simulink model "SMES_DC_STEP_1170KW_1000V_0"  (R2020a)
settings: Solver=VariableStepAuto  StartTime=0.0  StopTime=2  RelTol=1e-3
InitFcn:
  | Timer= 1e-3
StartFcn:
  | Timer= 1e-3
undefined symbols (not defined in the file): L
libraries: powerlib x33, simulink x5, powerlib_meascontrol x4
settings Model: Creator=JGC  LastModifiedBy=AGP
settings DataIOCC: ReturnWorkspaceOutputs=off

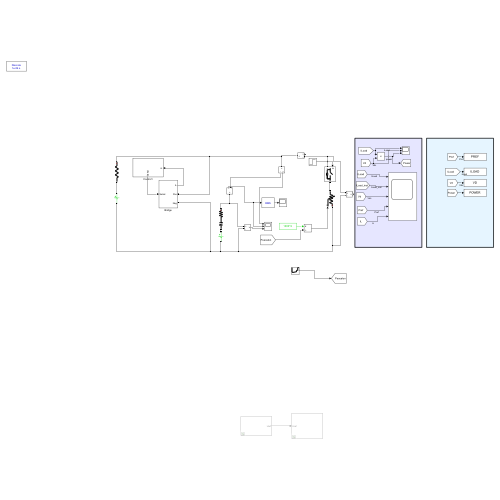
[thumbnail: Simulink's stored preview of the top-level diagram]
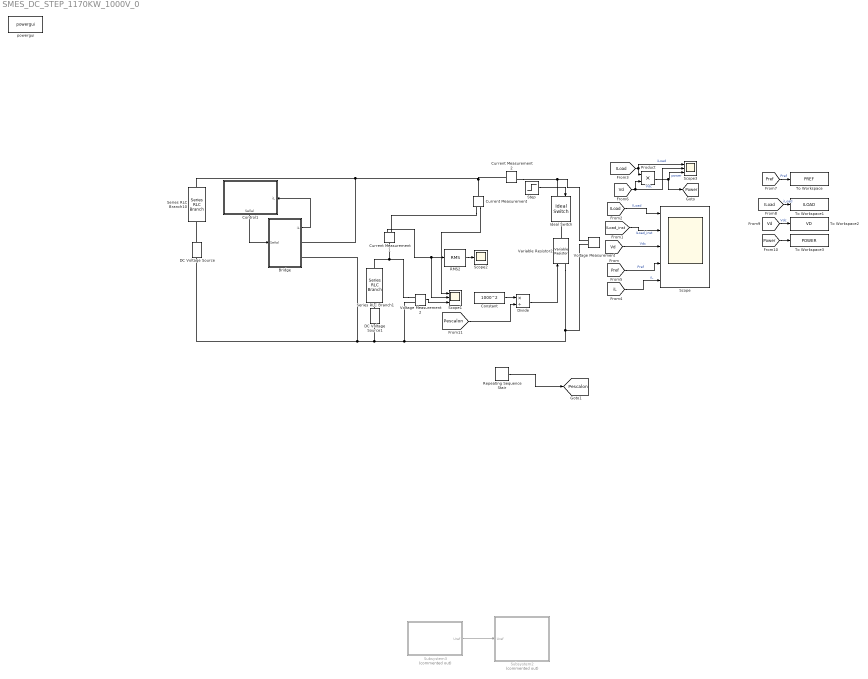
== system SMES_DC_STEP_1170KW_1000V_0 ==
  Bridge : Subsystem
  Constant : Constant  Value=1000^2
  Control1 : Subsystem
      settings: PortSchema="{\"entries\":[{\"content\":{\"sides\":[{\"content\":{},\"type\":\"ConnectorPlacement.EquallySpacedRectSide\",\"uuid\":\"048239fd-db1d-471e-8dcc-44b0bb6d6223\"},{\"content\":{\"connectorIds\":[\"In1\"],\"side\":\"RIGHT\"},\"type\":\"ConnectorPlacement.EquallySpacedRectSide\",\"uuid\":\"9151a5a4-d268-441e-9897-4ef179ef940a\"},{\"content\":{\"side\":\"TOP\"},\"type\":\"ConnectorPlacement.EquallySpacedRectSide\",\"uuid\":\"4fbf07e4-6277-4577-bdb6-c05e0e5af188\"},{\"content\":{\"connectorIds\":[\"Out1\"],\"side\":\"BOTTOM\"},\"type\":\"ConnectorPlacement.EquallySpacedRectSide\",\"uuid\":\"b1bdda97-6966-4786-9e6a-4bb3780cee9c\"}]},\"type\":\"ConnectorPlacement.EquallySpacedConnector\",\"uuid\":\"ea29d1f9-a328-47e5-9b19-c2665d8c639d\"}],\"packageUris\":[\"http://schema.mathworks.com/mf0/Connector/R2020b\"],\"version\":\"1.0\"}"
  Current Measurement : powerlib/Measurements/Current Measurement  PhasorSimulation=off  OutputType=Complex  PSBequivalent=0
  Current Measurement1 : powerlib/Measurements/Current Measurement  PhasorSimulation=off  OutputType=Complex  PSBequivalent=0
  Current Measurement2 : powerlib/Measurements/Current Measurement  PhasorSimulation=off  OutputType=Complex  PSBequivalent=0
  DC Voltage Source : powerlib/Electrical Sources/DC Voltage Source  Amplitude=1000  Measurements=None
  DC Voltage Source1 : powerlib/Electrical Sources/DC Voltage Source  Amplitude=1000  Measurements=None
  Divide : Product  Inputs=*/
  Ideal Switch : powerlib/Power Electronics/Ideal Switch  Ron=0.001  Lon=0  IC=0  Rs=1e5  Cs=inf  Measurements=off
  Product : Product
  RMS2 : powerlib_meascontrol/Measurements/RMS  TrueRMS=on  Freq=50  RMSInit=0  Ts=0
  Repeating Sequence Stair : simulink/Sources/Repeating Sequence Stair  OutValues=[35e3 50e3 100e3 175e3 500e3 1170e3].'  tsamp=0.2  OutMin=[]  OutMax=[]  OutDataTypeStr=double  OutputDataTypeScalingMode=double  OutDataType=fixdt(0,8)  ConRadixGroup=Best Precision: Vector-wise  OutScaling=2^-12
  Scope : Scope  NumInputPorts=5
  Scope1 : Scope  NumInputPorts=3
  Scope2 : Scope
  Scope3 : Scope  NumInputPorts=3
  Series RLC Branch1 : powerlib/Elements/Series RLC Branch  LConnTagsString=__new0  RConnTagsString=__new0  BranchType=RC  Resistance=0.15e-3*200  Inductance=L  SetiL0=off  InitialCurrent=0  Capacitance=3400/200  Setx0=off  InitialVoltage=800  Measurements=None
  Series RLC Branch10 : powerlib/Elements/Series RLC Branch  LConnTagsString=__new0  RConnTagsString=__new0  BranchType=R  Resistance=1e-2  Inductance=L  SetiL0=off  InitialCurrent=0  Capacitance=1e-3  Setx0=off  InitialVoltage=800  Measurements=None
  Step : Step  Time=0.01  SampleTime=0
  Subsystem2 : Subsystem  Commented=on
  Subsystem3 : Subsystem  Commented=on
  To Workspace : ToWorkspace  VariableName=PREF  SaveFormat=Structure With Time  SampleTime=Timer
  To Workspace1 : ToWorkspace  VariableName=ILOAD  SaveFormat=Structure With Time  SampleTime=Timer
  To Workspace2 : ToWorkspace  VariableName=VD  SaveFormat=Structure With Time  SampleTime=Timer
  To Workspace3 : ToWorkspace  VariableName=POWER  SaveFormat=Structure With Time  SampleTime=Timer
  Variable Resistor2 : powerlib/Elements/Variable Resistor  Rabsmin=1e-3
  Voltage Measurement : powerlib/Measurements/Voltage Measurement  PhasorSimulation=off  OutputType=Complex  PSBequivalent=0
  Voltage Measurement2 : powerlib/Measurements/Voltage Measurement  PhasorSimulation=off  OutputType=Complex  PSBequivalent=0
  powergui : powerlib/powergui  Priority=1  SimulationMode=Discrete  SampleTime=1e-6  frequency=60  Iterations=50  frequencyindice=0  Pbase=100e6  ErrMax=1e-4  UnitsV=kV  UnitsW=MW  buscounter=0  FunctionMessages=off  echomessages=off  EnableUseOfTLC=off  CurrentSourceSwitches=off  DisableSnubberDevices=off  DisableRonSwitches=off  DisableVfSwitches=off  DisplayEquations=off  AutomaticDiscreteSolvers=off  SolverType=Tustin/Backward Euler (TBE)  Interpol=off  ExternalGateDelay=off  methode=off  Ts=100  x0status=zero  SPID=off  SwTol=0  HookPort=off  NonlinearTolerance=1e-4  nMaxIteration=100  ContinueOnMaxIteration=off  RestoreLinks=warning  ResistiveCurrentMeasurement=off  Frange=[0:2:500]  Ylog=off  Xlog=on  ShowGrid=off  save=off  variable=ZData  structure=0  ZoomFFT=off  StartTime=0.0  cycles=1  DisplayStyle=1  fundamental=60  FreqAxis=off  MaxFrequency=1000  frequencyindicesteady=1  RmsSteady=1  display=off
  tag scope: Pescalon=global, Power=global
  wires:
  Step/1 -> Ideal Switch/1
  [Pref] -> Scope/4  "Pref"
  Current Measurement/1 -> Scope1/1
  Subsystem3/1(Uref) -> Subsystem2/1(Uref)
  [iL] -> Scope/5  "iL"
  [ILoad_inst] -> Scope/2  "ILoad_inst"
  [ILoad] -> Scope/1  "ILoad"
  [Vd] -> Scope/3  "Vdc"
  Control1/1("Señal ") -> Bridge/1(Señal)
  Bridge/1(iL) -> Control1/1(iL)
  Current Measurement1/1 -> Scope1/2, RMS2/1
  Voltage Measurement2/1 -> Scope1/3
  RMS2/1 -> Scope2/1
  [Pescalon] -> Divide/2
  Divide/1 -> Variable Resistor2/1
  Constant/1 -> Divide/1
  [ILoad] -> Product/1, Scope3/1  "iLoad"
  Product/1 -> [Power], Scope3/3  "power"
  [Vd] -> Product/2, Scope3/2  "Vdc"
  [Pref] -> To Workspace/1  "Pref"
  [ILoad] -> To Workspace1/1  "iLoad"
  [Vd] -> To Workspace2/1  "Vdc"
  [Power] -> To Workspace3/1
  Repeating Sequence Stair/1 -> [Pescalon]
  connections:
  DC Voltage Source/RConn1 -- Series RLC Branch10/RConn1
  Current Measurement/RConn1 -- Current Measurement1/RConn1
  Variable Resistor2/RConn1 -- Ideal Switch/RConn1
  Ideal Switch/LConn1 -- Current Measurement2/RConn1 -- Voltage Measurement/LConn1
  Bridge/RConn2 -- DC Voltage Source/LConn1 -- DC Voltage Source1/LConn1 -- Voltage Measurement/LConn2 -- Variable Resistor2/LConn1 -- Voltage Measurement2/LConn2
  Voltage Measurement2/LConn1 -- Series RLC Branch1/LConn1 -- Current Measurement1/LConn1
  DC Voltage Source1/RConn1 -- Series RLC Branch1/RConn1
  Current Measurement/LConn1 -- Current Measurement2/LConn1 -- Bridge/RConn1 -- Series RLC Branch10/LConn1

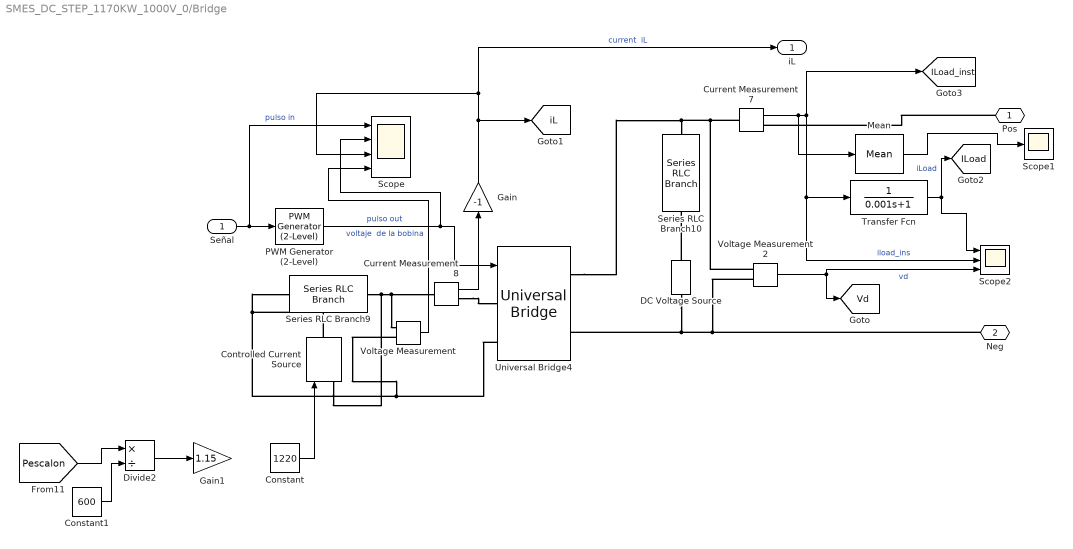
== system SMES_DC_STEP_1170KW_1000V_0/Bridge ==
  Señal : Inport
  Constant : Constant  Value=1220
  Constant1 : Constant  Value=600
  Controlled Current Source : powerlib/Electrical Sources/Controlled Current Source  Initialize=on  Source_Type=AC  Amplitude=0  Phase=0  Frequency=0  Measurements=None
  Current Measurement7 : powerlib/Measurements/Current Measurement  PhasorSimulation=off  OutputType=Complex  PSBequivalent=0
  Current Measurement8 : powerlib/Measurements/Current Measurement  PhasorSimulation=off  OutputType=Complex  PSBequivalent=0
  DC Voltage Source : powerlib/Electrical Sources/DC Voltage Source  Amplitude=1000  Measurements=None
  Divide2 : Product  Inputs=*/
  Gain : Gain  Gain=-1
  Gain1 : Gain  Gain=1.15
  Mean : powerlib_meascontrol/Measurements/Mean  Freq=60  Vinit=0  Ts=0
  PWM Generator (2-Level) : powerlib_meascontrol/Pulse & Signal Generators/PWM Generator (2-Level)  ModulatorType=Single-phase full-bridge (4 pulses)  ModulatorMode=Unsynchronized  Fc=40*50  Pc=90  nF=27  MinMax="[ -1  1 ]"  SamplingTechnique=Natural  ModulatingSignals=off  m=0.8  Freq=60  Phase=0  Ts=0  ShowCarrierOutport=off
  Scope : Scope  NumInputPorts=4
  Scope1 : Scope
  Scope2 : Scope  NumInputPorts=3
  Series RLC Branch10 : powerlib/Elements/Series RLC Branch  LConnTagsString=__new0  RConnTagsString=__new0  BranchType=RC  Resistance=1e-1  Inductance=L  SetiL0=off  InitialCurrent=0  Capacitance=1e-3  Setx0=off  InitialVoltage=800  Measurements=None
  Series RLC Branch9 : powerlib/Elements/Series RLC Branch  LConnTagsString=__new0  RConnTagsString=__new0  BranchType=RL  Resistance=0.1  Inductance=5.42  SetiL0=off  InitialCurrent=0  Capacitance=1e-3  Setx0=off  InitialVoltage=0  Measurements=None
  Transfer Fcn : TransferFcn  Denominator=[0.001 1]
  Universal Bridge4 : powerlib/Power Electronics/Universal Bridge  Arms=2  SnubberResistance=1e5  SnubberCapacitance=inf  Device=IGBT / Diodes  Ron=1e-3  Lon=0  ForwardVoltages="[  1  1  ]"  ForwardVoltage=0  GTOparameters=[ 10e-6 , 20e-6 ]  IGBTparameters=[ 1e-6 , 2e-6 ]  Measurements=None  Measurements_2=None  converterType=Rectifier
  Voltage Measurement : powerlib/Measurements/Voltage Measurement  PhasorSimulation=off  OutputType=Complex  PSBequivalent=0
  Voltage Measurement2 : powerlib/Measurements/Voltage Measurement  PhasorSimulation=off  OutputType=Complex  PSBequivalent=0
  Pos : PMIOPort  Side=Right
  Neg : PMIOPort  Port=2  Side=Right
  iL : Outport
  tag scope: ILoad=global, ILoad_inst=global, Vd=global, iL=global
  wires:
  Gain/1 -> Scope/3, iL/1, [iL]  "current \tiL"
  PWM Generator (2-Level)/1 -> Scope/2, Universal Bridge4/1  "pulso out"
  Current Measurement8/1 -> Gain/1
  Señal/1 -> Scope/1, PWM Generator (2-Level)/1  "pulso in"
  Transfer Fcn/1 -> [ILoad], Scope2/1  "iLoad"
  Current Measurement7/1 -> Mean/1, Scope2/2, Transfer Fcn/1, [ILoad_inst]  "iload_ins"
  Voltage Measurement/1 -> Scope/4  "voltaje  de la bobina"
  Voltage Measurement2/1 -> [Vd], Scope2/3  "vd"
  Mean/1 -> Scope1/1
  Constant1/1 -> Divide2/2
  [Pescalon] -> Divide2/1
  Divide2/1 -> Gain1/1
  Constant/1 -> Controlled Current Source/1
  connections:
  Neg/RConn1 -- Voltage Measurement2/LConn2 -- DC Voltage Source/LConn1 -- Universal Bridge4/RConn2
  Current Measurement8/RConn1 -- Universal Bridge4/LConn1
  Universal Bridge4/LConn2 -- Voltage Measurement/LConn2 -- Controlled Current Source/RConn1 -- Series RLC Branch9/LConn1
  Voltage Measurement2/LConn1 -- Universal Bridge4/RConn1 -- Series RLC Branch10/LConn1 -- Current Measurement7/LConn1
  DC Voltage Source/RConn1 -- Series RLC Branch10/RConn1
  Pos/RConn1 -- Current Measurement7/RConn1
  Series RLC Branch9/RConn1 -- Current Measurement8/LConn1 -- Voltage Measurement/LConn1 -- Controlled Current Source/LConn1

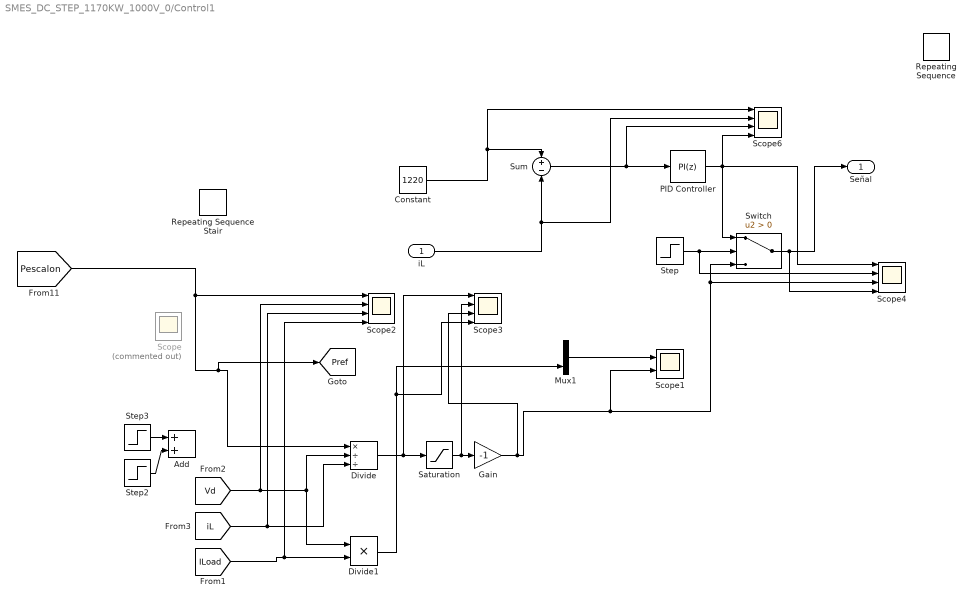
== system SMES_DC_STEP_1170KW_1000V_0/Control1 ==
  iL : Inport
  Add : Sum
  Constant : Constant  Value=1220
  Divide : Product  Inputs=*//
  Divide1 : Product  Inputs=**
  Gain : Gain  Gain=-1
  Mux1 : Mux  Inputs=2
  PID Controller : simulink/Continuous/PID Controller  Controller=PI  Form=Parallel  TimeDomain=Discrete-time  UseExternalTs=off  SampleTime=2.5e-4  IntegratorMethod=Forward Euler  ControllerParametersSource=internal  P=1  I=0.1  D=0  N=100  UseFilter=on  TunerSelectOption=Transfer Function Based (PID Tuner App)  InitialConditionSource=internal  InitialConditionForIntegrator=0  InitialConditionForFilter=0  DifferentiatorICPrevScaledInput=0  ExternalReset=none  TrackingMode=off  Kt=1  LimitOutput=on  UpperSaturationLimit=1  LowerSaturationLimit=-1  LinearizeAsGain=on  AntiWindupMode=clamping  Kb=1  POutMin=[]  POutMax=[]  IOutMin=[]  IOutMax=[]  DOutMin=[]  DOutMax=[]  NOutMin=[]  NOutMax=[]  SumOutMin=[]  SumOutMax=[]  SaturationOutMin=[]  SaturationOutMax=[]  PParamMin=[]  PParamMax=[]  IParamMin=[]  IParamMax=[]  DParamMin=[]  DParamMax=[]  NParamMin=[]  NParamMax=[]  KbParamMin=[]  KbParamMax=[]  KtParamMin=[]  KtParamMax=[]  KbOutMin=[]  KbOutMax=[]  KtOutMin=[]  KtOutMax=[]  IntegratorOutMin=[]  IntegratorOutMax=[]  FilterOutMin=[]  FilterOutMax=[]  SumI1OutMin=[]  SumI1OutMax=[]  SumI2OutMin=[]  SumI2OutMax=[]  SumI3OutMin=[]  SumI3OutMax=[]  SumI4OutMin=[]  SumI4OutMax=[]  SumDOutMin=[]  SumDOutMax=[]  DifferentiatorOutMin=[]  DifferentiatorOutMax=[]  FilterDiffOutCoefMin=[]  FilterDiffOutCoefMax=[]  ReciprocalOutMin=[]  ReciprocalOutMax=[]  SumDenOutMin=[]  SumDenOutMax=[]  SumNumOutMin=[]  SumNumOutMax=[]  DivideOutMin=[]  DivideOutMax=[]  UdiffTsProdOutMin=[]  UdiffTsProdOutMax=[]  NTsProdOutMin=[]  NTsProdOutMax=[]  UintegralTsProdOutMin=[]  UintegralTsProdOutMax=[]  UngainTsProdOutMin=[]  UngainTsProdOutMax=[]  IntegratorContinuousStateAttributes=''  IntegratorStateMustResolveToSignalObject=off  IntegratorRTWStateStorageClass=Auto  FilterContinuousStateAttributes=''  FilterStateMustResolveToSignalObject=off  FilterRTWStateStorageClass=Auto  ParallelPVariant=InternalParameters  IdealPVariant=Disabled  IVariant=InternalParameters  DVariant=Disabled  IntegratorVariant=Discrete  SatVariant=Enabled  AWVariant=DiscClampingParallel  PCopyVariant=Disabled  TRVariant=Disabled  FdbkBlocksVariant=Forward  IdealPFdbkVariant=Disabled  SatFdbkVariant=Disabled  DerivativeFilterVariant=Disabled  NVariant=Disabled  NCopyVariant=Disabled_SignalSpec  FilterICVariant=Disabled  IntegratorICVariant=InternalICs  ExternalResetVariant=Disabled  TRSumVariant=Passthrough  SumFdbkVariant=Disabled  SumVariant=Sum_PI  TsampFilterVariant=InternalTs  TsampNgainVariant=Passthrough  TsampIntegralVariant=Disabled_SignalSpec
  Repeating Sequence : simulink/Sources/Repeating Sequence  rep_seq_t=[0 0.001 0.2 0.201 0.4 0.401 0.6 0.601 0.8 0.801 1 1.001]  rep_seq_y=[1 0 1 0 1 0 1 0 1 0 1 0]
  Repeating Sequence Stair : simulink/Sources/Repeating Sequence Stair  OutValues=[0 5e4 -5e4 ].'  tsamp=5e-3  OutMin=[]  OutMax=[]  OutDataTypeStr=double  OutputDataTypeScalingMode=double  OutDataType=fixdt(0,8)  ConRadixGroup=Best Precision: Vector-wise  OutScaling=2^-12
  Saturation : Saturate  UpperLimit=1  LowerLimit=-1
  Scope : Scope  Commented=on
  Scope1 : Scope  NumInputPorts=2
  Scope{2..4,6} (4 alike) : Scope  NumInputPorts=4
  Step : Step  Time=0.001  Before=1  After=0  SampleTime=0
  Step2 : Step  Time=0.006  After=-100000  SampleTime=0
  Step3 : Step  Time=0.002  After=50000  SampleTime=0
  Sum : Sum  Inputs=+-
  Switch : Switch  Criteria=u2 > Threshold
  "Señal " : Outport  VectorParamsAs1DForOutWhenUnconnected=off
  tag scope: Pref=global
  wires:
  Constant/1 -> Scope6/1, Sum/1
  iL/1 -> Scope6/2, Sum/2
  Sum/1 -> Scope6/3, PID Controller/1
  Switch/1 -> Scope4/4, "Señal "/1
  Gain/1 -> Scope3/3, Scope4/3, Switch/3, Scope1/2
  Step/1 -> Scope4/2, Switch/2
  [ILoad] -> Scope2/4, Divide1/2
  Saturation/1 -> Scope3/2, Gain/1
  [iL] -> Scope2/3, Divide/3
  Divide1/1 -> Scope3/4, Mux1/2
  Divide/1 -> Scope3/1, Saturation/1
  Mux1/1 -> Scope1/1
  [Vd] -> Scope2/2, Divide1/1, Divide/2
  Step3/1 -> Add/1
  Step2/1 -> Add/2
  [Pescalon] -> [Pref], Divide/1, Scope2/1
  PID Controller/1 -> Scope4/1, Switch/1, Scope6/4

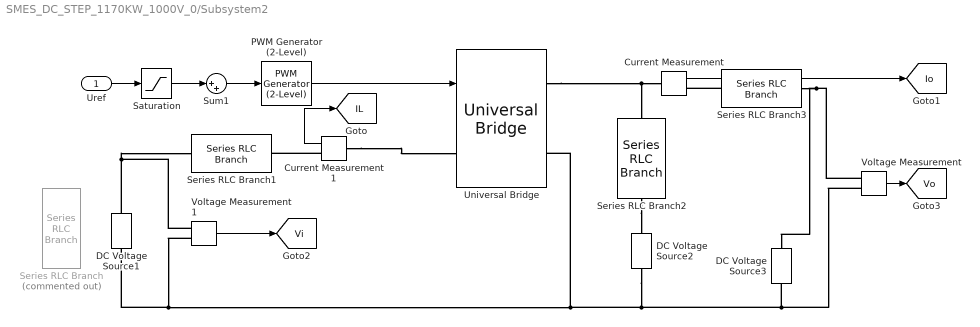
== system SMES_DC_STEP_1170KW_1000V_0/Subsystem2 ==
  Uref : Inport
  Current Measurement : powerlib/Measurements/Current Measurement  PhasorSimulation=off  OutputType=Complex  PSBequivalent=0
  Current Measurement1 : powerlib/Measurements/Current Measurement  PhasorSimulation=off  OutputType=Complex  PSBequivalent=0
  DC Voltage Source1 : powerlib/Electrical Sources/DC Voltage Source  Amplitude=1250  Measurements=None
  DC Voltage Source2 : powerlib/Electrical Sources/DC Voltage Source  Amplitude=2500  Measurements=None
  DC Voltage Source3 : powerlib/Electrical Sources/DC Voltage Source  Amplitude=2500  Measurements=None
  PWM Generator (2-Level) : powerlib_meascontrol/Pulse & Signal Generators/PWM Generator (2-Level)  ModulatorType=Single-phase half-bridge (2 pulses)  ModulatorMode=Unsynchronized  Fc=60*60  Pc=0  nF=27  MinMax="[-1  1 ]"  SamplingTechnique=Natural  ModulatingSignals=off  m=0.8  Freq=60  Phase=0  Ts=1e-6  ShowCarrierOutport=off
  Saturation : Saturate  UpperLimit=1  LowerLimit=-1
  Series RLC Branch : powerlib/Elements/Series RLC Branch  Commented=on  LConnTagsString=__new0  RConnTagsString=__new0  BranchType=RC  Resistance=1e-3  Inductance=1e-3  SetiL0=off  InitialCurrent=0  Capacitance=2337.8  Setx0=on  InitialVoltage=1800  Measurements=None
  Series RLC Branch1 : powerlib/Elements/Series RLC Branch  LConnTagsString=__new0  RConnTagsString=__new0  BranchType=L  Resistance=1  Inductance=3e-3  SetiL0=on  InitialCurrent=0  Capacitance=1e-6  Setx0=off  InitialVoltage=0  Measurements=None
  Series RLC Branch2 : powerlib/Elements/Series RLC Branch  LConnTagsString=__new0  RConnTagsString=__new0  BranchType=RC  Resistance=1e-3  Inductance=1e-3  SetiL0=off  InitialCurrent=0  Capacitance=1e-3  Setx0=off  InitialVoltage=0  Measurements=None
  Series RLC Branch3 : powerlib/Elements/Series RLC Branch  LConnTagsString=__new0  RConnTagsString=__new0  BranchType=RL  Resistance=1  Inductance=10e-6  SetiL0=on  InitialCurrent=0  Capacitance=1e-6  Setx0=off  InitialVoltage=0  Measurements=None
  Sum1 : Sum  Inputs=|++
  Universal Bridge : powerlib/Power Electronics/Universal Bridge  Arms=1  SnubberResistance=1e5  SnubberCapacitance=inf  Device=IGBT / Diodes  Ron=1e-3  Lon=0  ForwardVoltages="[  0  0  ]"  ForwardVoltage=0  GTOparameters=[ 10e-6 , 20e-6 ]  IGBTparameters=[ 1e-6 , 2e-6 ]  Measurements=None  Measurements_2=None  converterType=Rectifier
  Voltage Measurement : powerlib/Measurements/Voltage Measurement  PhasorSimulation=off  OutputType=Complex  PSBequivalent=0
  Voltage Measurement1 : powerlib/Measurements/Voltage Measurement  PhasorSimulation=off  OutputType=Complex  PSBequivalent=0
  tag scope: IL=global, Io=global, Vi=global, Vo=global
  wires:
  Uref/1 -> Saturation/1
  Voltage Measurement/1 -> [Vo]
  Current Measurement/1 -> [Io]
  Voltage Measurement1/1 -> [Vi]
  Current Measurement1/1 -> [IL]
  PWM Generator (2-Level)/1 -> Universal Bridge/1
  Saturation/1 -> Sum1/1
  Sum1/1 -> PWM Generator (2-Level)/1
  connections:
  Voltage Measurement/LConn2 -- DC Voltage Source3/LConn1 -- DC Voltage Source2/LConn1 -- DC Voltage Source1/LConn1 -- Voltage Measurement1/LConn2 -- Universal Bridge/RConn2
  Universal Bridge/RConn1 -- Current Measurement/LConn1 -- Series RLC Branch2/LConn1
  Voltage Measurement/LConn1 -- DC Voltage Source3/RConn1 -- Series RLC Branch3/RConn1
  Voltage Measurement1/LConn1 -- Series RLC Branch1/LConn1 -- DC Voltage Source1/RConn1
  Current Measurement1/LConn1 -- Universal Bridge/LConn1
  Current Measurement1/RConn1 -- Series RLC Branch1/RConn1
  Series RLC Branch2/RConn1 -- DC Voltage Source2/RConn1
  Series RLC Branch3/LConn1 -- Current Measurement/RConn1

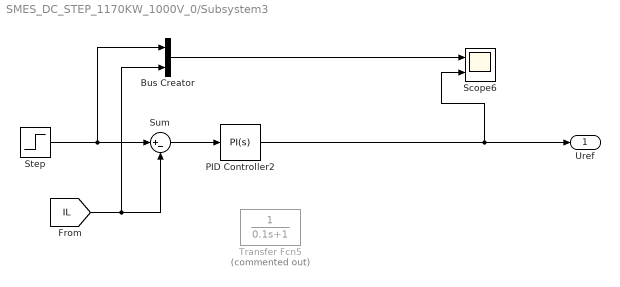
== system SMES_DC_STEP_1170KW_1000V_0/Subsystem3 ==
  Bus Creator : BusCreator  Inputs=2
  PID Controller2 : simulink/Continuous/PID Controller  Controller=PI  Form=Parallel  TimeDomain=Continuous-time  UseExternalTs=off  SampleTime=-1  IntegratorMethod=Forward Euler  ControllerParametersSource=internal  P=0.02  I=0.02  D=0.01  N=100  UseFilter=on  TunerSelectOption=Transfer Function Based (PID Tuner App)  InitialConditionSource=internal  InitialConditionForIntegrator=0  InitialConditionForFilter=0  DifferentiatorICPrevScaledInput=0  ExternalReset=none  TrackingMode=off  Kt=1  LimitOutput=off  UpperSaturationLimit=1  LowerSaturationLimit=0  LinearizeAsGain=on  AntiWindupMode=none  Kb=1  POutMin=[]  POutMax=[]  IOutMin=[]  IOutMax=[]  DOutMin=[]  DOutMax=[]  NOutMin=[]  NOutMax=[]  SumOutMin=[]  SumOutMax=[]  SaturationOutMin=[]  SaturationOutMax=[]  PParamMin=[]  PParamMax=[]  IParamMin=[]  IParamMax=[]  DParamMin=[]  DParamMax=[]  NParamMin=[]  NParamMax=[]  KbParamMin=[]  KbParamMax=[]  KtParamMin=[]  KtParamMax=[]  KbOutMin=[]  KbOutMax=[]  KtOutMin=[]  KtOutMax=[]  IntegratorOutMin=[]  IntegratorOutMax=[]  FilterOutMin=[]  FilterOutMax=[]  SumI1OutMin=[]  SumI1OutMax=[]  SumI2OutMin=[]  SumI2OutMax=[]  SumI3OutMin=[]  SumI3OutMax=[]  SumI4OutMin=[]  SumI4OutMax=[]  SumDOutMin=[]  SumDOutMax=[]  DifferentiatorOutMin=[]  DifferentiatorOutMax=[]  FilterDiffOutCoefMin=[]  FilterDiffOutCoefMax=[]  ReciprocalOutMin=[]  ReciprocalOutMax=[]  SumDenOutMin=[]  SumDenOutMax=[]  SumNumOutMin=[]  SumNumOutMax=[]  DivideOutMin=[]  DivideOutMax=[]  UdiffTsProdOutMin=[]  UdiffTsProdOutMax=[]  NTsProdOutMin=[]  NTsProdOutMax=[]  UintegralTsProdOutMin=[]  UintegralTsProdOutMax=[]  UngainTsProdOutMin=[]  UngainTsProdOutMax=[]  IntegratorContinuousStateAttributes=''  IntegratorStateMustResolveToSignalObject=off  IntegratorRTWStateStorageClass=Auto  FilterContinuousStateAttributes=''  FilterStateMustResolveToSignalObject=off  FilterRTWStateStorageClass=Auto  ParallelPVariant=InternalParameters  IdealPVariant=Disabled  IVariant=InternalParameters  DVariant=Disabled  IntegratorVariant=Continuous  SatVariant=Disabled  AWVariant=Passthrough  PCopyVariant=Disabled  TRVariant=Disabled  FdbkBlocksVariant=Forward  IdealPFdbkVariant=Disabled  SatFdbkVariant=Disabled  DerivativeFilterVariant=Disabled  NVariant=Disabled  NCopyVariant=Disabled_SignalSpec  FilterICVariant=Disabled  IntegratorICVariant=InternalICs  ExternalResetVariant=Disabled  TRSumVariant=Passthrough  SumFdbkVariant=Disabled  SumVariant=Sum_PI  TsampFilterVariant=InternalTs  TsampNgainVariant=Passthrough  TsampIntegralVariant=Disabled_SignalSpec
  Scope6 : Scope  NumInputPorts=2
  Step : Step  Time=0.2  After=1000  SampleTime=0
  Sum : Sum  Inputs=|+-
  Transfer Fcn5 : TransferFcn  Commented=on  Denominator=[0.1 1]
  Uref : Outport
  wires:
  Sum/1 -> PID Controller2/1
  [IL] -> Bus Creator/2, Sum/2
  Bus Creator/1 -> Scope6/1
  Step/1 -> Bus Creator/1, Sum/1
  PID Controller2/1 -> Scope6/2, Uref/1
